simulink model "Chevrolet_PHEVmodel"  (R2024b)
settings: Solver=VariableStepAuto  StartTime=0.0  StopTime=10.0  RelTol=1e-3
undefined symbols (not defined in the file): automatic_gearbox, DiscIntNeverNeededParam, eta_EG_map, eta_EM_map, g, h, H_u, k_cs, P_aux, P_CE_cutoff, P_CE_idle, r, rho, rho_f, T_CE_cutoff, T_CE_max, T_EG_max, T_EM_max, theta_CE, theta_EM, V_CE_map, w_CE_idle, w_CE_max, w_CE_upper, w_EG_row, w_EG_upper, w_EM_row, w_EM_upper
(part 2 of 2)

== system Chevrolet_PHEVmodel/Automatic Gear Box1/Power flow/Wheel -> Engine ==
  w_wheel : Inport
  T_wheel : Inport  Port=2
  gear : Inport  Port=3
  Constant1 : Constant  Value=P_GT0
  Constant2 : Constant  Value=inf
  Gain1 : Gain  Gain=e_GT  SaturateOnIntegerOverflow=on  OutDataTypeStr=Inherit: Same as input  ParamDataTypeStr=Inherit: Same as input
  Gain2 : Gain  Gain=1/e_GT  SaturateOnIntegerOverflow=on  OutDataTypeStr=Inherit: Same as input  ParamDataTypeStr=Inherit: Same as input
  Product2 : Product  Inputs=*/  InputSameDT=on  RndMeth=Zero  SaturateOnIntegerOverflow=on  OutDataTypeStr=Inherit: Same as first input
  Product3 : Product  Inputs=/*  InputSameDT=on  RndMeth=Zero  SaturateOnIntegerOverflow=on  OutDataTypeStr=Inherit: Same as first input
  Sum : Sum  InputSameDT=on  SaturateOnIntegerOverflow=on  OutDataTypeStr=Inherit: Same as first input
  Switch1 : Switch  Threshold=w_wheel_min
  T_MGB- : Outport  InitialOutput=0
  wires:
  w_wheel/1 -> Switch1/1, Switch1/2
  gear/1 -> Gain2/1
  Constant2/1 -> Switch1/3
  Switch1/1 -> Gain1/1
  Constant1/1 -> Product3/2
  Gain2/1 -> Product2/2
  Product2/1 -> T_MGB-/1
  Product3/1 -> Sum/2
  Sum/1 -> Product2/1
  Gain1/1 -> Product3/1
  T_wheel/1 -> Sum/1

== system Chevrolet_PHEVmodel/PHEV Battery/Cell electrical model/State of charge calculation ==
  I_cell [A] : Inport
  Rt_initSOC [-] : Inport  Port=2
  Constant1 : Constant
  Constant2 : Constant  Value=35
  Constant4 : Constant  Value=3600
  Discrete-Time Integrator : DiscreteIntegrator  InitialConditionSource=external  ICPrevOutput=DiscIntNeverNeededParam  ICPrevScaledInput=DiscIntNeverNeededParam
  Product : Product  Inputs=*/  OutMin=-500  OutMax=500  RndMeth=Zero
  Product1 : Product  Inputs=*/  RndMeth=Zero
  Sum : Sum  Inputs=|-+
  Rt_SOC [-] : Outport
  Rt_DOD [-] : Outport  Port=2
  wires:
  I_cell [A]/1 -> Product/1
  Product/1 -> Product1/1
  Constant2/1 -> Product1/2
  Product1/1 -> Discrete-Time Integrator/1
  Discrete-Time Integrator/1 -> Sum/1, Rt_SOC [-]/1
  Sum/1 -> Rt_DOD [-]/1
  Constant4/1 -> Product/2
  Constant1/1 -> Sum/2
  Rt_initSOC [-]/1 -> Discrete-Time Integrator/2

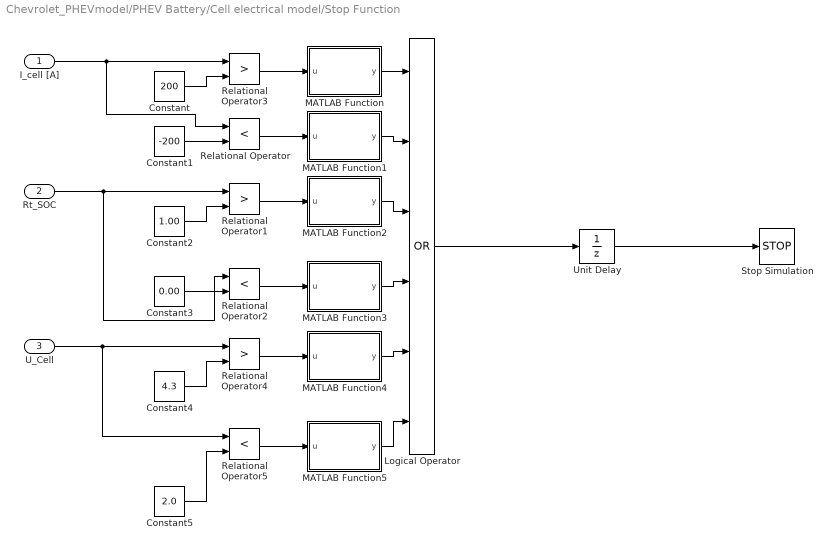
== system Chevrolet_PHEVmodel/PHEV Battery/Cell electrical model/Stop Function ==
  I_cell [A] : Inport
  Rt_SOC : Inport  Port=2
  U_Cell : Inport  Port=3
  Constant : Constant  Value=200
  Constant1 : Constant  Value=-200
  Constant2 : Constant  Value=1.00
  Constant3 : Constant  Value=0.00
  Constant4 : Constant  Value=4.3
  Constant5 : Constant  Value=2.0
  Logical Operator : Logic  Operator=OR  Inputs=6  AllPortsSameDT=off  OutDataTypeStr=boolean
  MATLAB Function : MATLAB Function  TreatAsAtomicUnit=on
  MATLAB Function1 : MATLAB Function  TreatAsAtomicUnit=on
  MATLAB Function2 : MATLAB Function  TreatAsAtomicUnit=on
  MATLAB Function3 : MATLAB Function  TreatAsAtomicUnit=on
  MATLAB Function4 : MATLAB Function  TreatAsAtomicUnit=on
  MATLAB Function5 : MATLAB Function  TreatAsAtomicUnit=on
  Relational Operator : RelationalOperator  Operator=<  OutDataTypeStr=boolean  InputSameDT=off
  Relational Operator1 : RelationalOperator  Operator=>  OutDataTypeStr=boolean  InputSameDT=off
  Relational Operator2 : RelationalOperator  Operator=<  OutDataTypeStr=boolean  InputSameDT=off
  Relational Operator3 : RelationalOperator  Operator=>  OutDataTypeStr=boolean  InputSameDT=off
  Relational Operator4 : RelationalOperator  Operator=>  OutDataTypeStr=boolean  InputSameDT=off
  Relational Operator5 : RelationalOperator  Operator=<  OutDataTypeStr=boolean  InputSameDT=off
  Stop Simulation : Stop
  Unit Delay : UnitDelay  SampleTime=-1  HasFrameUpgradeWarning=on
  wires:
  Rt_SOC/1 -> Relational Operator2/1, Relational Operator1/1
  I_cell [A]/1 -> Relational Operator/1, Relational Operator3/1
  U_Cell/1 -> Relational Operator5/1, Relational Operator4/1
  Constant/1 -> Relational Operator3/2
  Constant1/1 -> Relational Operator/2
  Constant2/1 -> Relational Operator1/2
  Constant3/1 -> Relational Operator2/2
  Constant5/1 -> Relational Operator5/2
  Constant4/1 -> Relational Operator4/2
  Logical Operator/1 -> Unit Delay/1
  Relational Operator3/1 -> MATLAB Function/1(u)
  Relational Operator/1 -> MATLAB Function1/1(u)
  Relational Operator1/1 -> MATLAB Function2/1(u)
  Relational Operator2/1 -> MATLAB Function3/1(u)
  Relational Operator4/1 -> MATLAB Function4/1(u)
  Relational Operator5/1 -> MATLAB Function5/1(u)
  MATLAB Function5/1(y) -> Logical Operator/6
  MATLAB Function4/1(y) -> Logical Operator/5
  MATLAB Function3/1(y) -> Logical Operator/4
  MATLAB Function2/1(y) -> Logical Operator/3
  MATLAB Function1/1(y) -> Logical Operator/2
  Unit Delay/1 -> Stop Simulation/1
  MATLAB Function/1(y) -> Logical Operator/1

== matlab function Chevrolet_PHEVmodel/PHEV Battery/Cell electrical model/Stop Function/MATLAB Function ==
  data: u input; y output
function y = fcn(u)
coder.extrinsic('sprintf')
coder.extrinsic('helpdlg')

if u == 1
helpdlg(sprintf('Battery Charge Current Too High'))
else
end
y = u;

== matlab function Chevrolet_PHEVmodel/Control Unit /MATLAB Function ==
  data: B_SoC input; y output; x_tot input; SoC_max input; SoC_min input; u_previous input
function y = fcn(B_SoC,x_tot,SoC_max,SoC_min,u_previous)
% Simple CDCS controller
if x_tot==1
    u = 0;
else
    if B_SoC > SoC_max
        u = 0;
    else
        if B_SoC < SoC_min
            u = 1;
        else
            u = u_previous;
        end
    end
end

y = u;

== matlab function Chevrolet_PHEVmodel/PHEV Battery/Cell electrical model/Stop Function/MATLAB Function1 ==
  data: u input; y output
function y = fcn(u)
coder.extrinsic('sprintf')
coder.extrinsic('helpdlg')

if u == 1
helpdlg(sprintf('High Battery Discharge Current'))
else
end
y = u;

== matlab function Chevrolet_PHEVmodel/PHEV Battery/Cell electrical model/Stop Function/MATLAB Function2 ==
  data: u input; y output
function y = fcn(u)
coder.extrinsic('sprintf')
coder.extrinsic('helpdlg')

if u == 1
helpdlg(sprintf('Upper SOC Limit'))
else
end
y = u;

== matlab function Chevrolet_PHEVmodel/PHEV Battery/Cell electrical model/Stop Function/MATLAB Function3 ==
  data: u input; y output
function y = fcn(u)
coder.extrinsic('sprintf')
coder.extrinsic('helpdlg')

if u == 1
helpdlg(sprintf('Lower SOC Limit'))
else
end
y = u;

== matlab function Chevrolet_PHEVmodel/PHEV Battery/Cell electrical model/Stop Function/MATLAB Function4 ==
  data: u input; y output
function y = fcn(u)
coder.extrinsic('sprintf')
coder.extrinsic('helpdlg')

if u == 1
helpdlg(sprintf('Cell Voltage Too High'))
else
end
y = u;

== matlab function Chevrolet_PHEVmodel/PHEV Battery/Cell electrical model/Stop Function/MATLAB Function5 ==
  data: u input; y output
function y = fcn(u)
coder.extrinsic('sprintf')
coder.extrinsic('helpdlg')

if u == 1
helpdlg(sprintf('Low Cell Voltage'))
else
end
y = u;
